simulink model "Without_Controller"  (R2020a)
settings: Solver=VariableStepAuto  StartTime=0.0  StopTime=30  RelTol=1e-3
libraries: powerlib x1
settings Model: Creator=Zebin  LastModifiedBy=Zebin

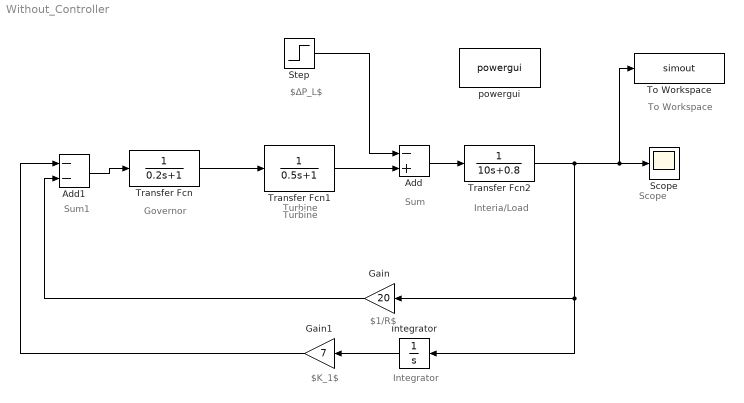
== system Without_Controller ==
  note: Sum
  note: Turbine
  note: Governor
  note: Sum1
  note: Interia/Load
  note: Scope
  note: To Workspace
  note: $ΔP_L$
  note: $1/R$
  note: Turbine
  note: Integrator
  note: $K_1$
  Add : Sum  Inputs=-+
  Add1 : Sum  Inputs=--
  Gain : Gain  Gain=20
  Gain1 : Gain  Gain=7
  Integrator : Integrator
  Scope : Scope
  Step : Step  Time=0  After=0.8  SampleTime=0
  To Workspace : ToWorkspace  VariableName=simout  SaveFormat=Timeseries  SampleTime=-1
  Transfer Fcn : TransferFcn  Denominator=[0.2 1]
  Transfer Fcn1 : TransferFcn  Denominator=[0.5 1]
  Transfer Fcn2 : TransferFcn  Denominator=[10 0.8]
  powergui : powerlib/powergui  Priority=1  SimulationMode=Continuous  SampleTime=50e-6  frequency=60  Iterations=50  frequencyindice=60  Pbase=100e6  ErrMax=1e-4  UnitsV=kV  UnitsW=MW  buscounter=0  FunctionMessages=off  echomessages=off  EnableUseOfTLC=off  CurrentSourceSwitches=off  DisableSnubberDevices=off  DisableRonSwitches=off  DisableVfSwitches=off  DisplayEquations=off  AutomaticDiscreteSolvers=off  SolverType=Tustin/Backward Euler (TBE)  Interpol=off  ExternalGateDelay=off  methode=off  Ts=100  x0status=blocks  SPID=on  SwTol=0  HookPort=off  NonlinearTolerance=1e-4  nMaxIteration=100  ContinueOnMaxIteration=off  RestoreLinks=warning  ResistiveCurrentMeasurement=off  Frange=[0:2:500]  Ylog=off  Xlog=on  ShowGrid=off  save=off  variable=ZData  structure=0  ZoomFFT=off  StartTime=0.0  cycles=1  DisplayStyle=1  fundamental=60  FreqAxis=off  MaxFrequency=1000  frequencyindicesteady=1  RmsSteady=1  display=off
  wires:
  Transfer Fcn/1 -> Transfer Fcn1/1
  Transfer Fcn1/1 -> Add/2
  Step/1 -> Add/1
  Transfer Fcn2/1 -> Integrator/1, Gain/1, To Workspace/1, Scope/1
  Add/1 -> Transfer Fcn2/1
  Add1/1 -> Transfer Fcn/1
  Integrator/1 -> Gain1/1
  Gain/1 -> Add1/2
  Gain1/1 -> Add1/1
